simulink model "ciagly_zlinearyzowany_model_dynamiczny"  (R2022b)
settings: Solver=VariableStepAuto  StartTime=0.0  StopTime=100  RelTol=1e-3
values from neighbouring files (symbols this model uses):
  a0 = data.a0    [Projekt1.m]    (also in wykresy_char_stat_nlin.m; wykresy_char_stat_zlin.m)
  a1 = data.a1    [Projekt1.m]    (also in wykresy_char_stat_nlin.m; wykresy_char_stat_zlin.m)
  a2 = data.a2    [Projekt1.m]    (also in wykresy_char_stat_nlin.m; wykresy_char_stat_zlin.m)
  alpha1 = data.alpha1    [Projekt1.m]    (also in wykresy_char_stat_nlin.m; wykresy_char_stat_zlin.m)
  alpha2 = data.alpha2    [Projekt1.m]    (also in wykresy_char_stat_nlin.m; wykresy_char_stat_zlin.m)
  alpha3 = data.alpha3    [Projekt1.m]    (also in wykresy_char_stat_nlin.m; wykresy_char_stat_zlin.m)
  alpha4 = data.alpha4    [Projekt1.m]    (also in wykresy_char_stat_nlin.m; wykresy_char_stat_zlin.m)
  b0 = data.b0    [Projekt1.m]    (also in wykresy_char_stat_nlin.m; wykresy_char_stat_zlin.m)
  t_u_step_sim = 1    [wykresy_char_dyn_dys.m]    (also in wykresy_char_dyn_zlin.m)
  u_step_sim = 1    [wykresy_char_dyn_dys.m]    (also in wykresy_char_dyn_zlin.m = u_step(j))
  ud = uds(i)    [wykresy_char_dyn_zlin.m]
  X_0 = [0;0;0]    [Projekt1.m]
settings Model: Creator=pioro  LastModifiedBy=pioro

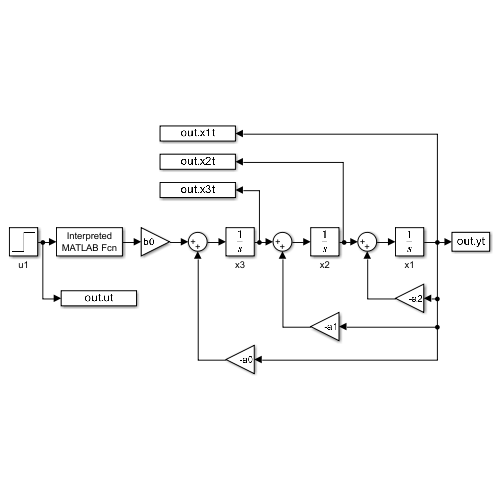
[thumbnail: Simulink's stored preview of the top-level diagram]
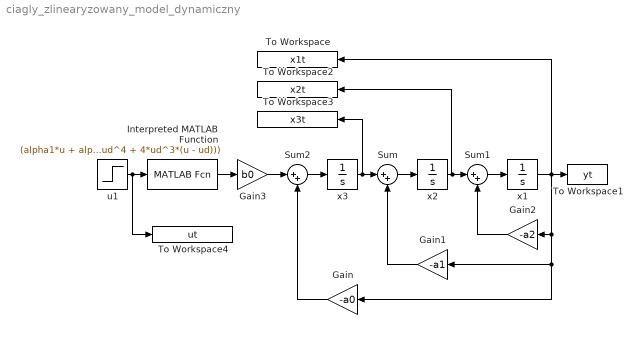
== system ciagly_zlinearyzowany_model_dynamiczny ==
  Gain : Gain  Gain=-a0
  Gain1 : Gain  Gain=-a1
  Gain2 : Gain  Gain=-a2
  Gain3 : Gain  Gain=b0
  Interpreted MATLAB Function : MATLABFcn  MATLABFcn=(alpha1*u + alpha2*(2*ud*(u - ud) + ud^2) + alpha3*(ud^3 + 3*ud^2*(u - ud)) + alpha4*(ud^4 + 4*ud^3*(u - ud)))
  Sum : Sum  Inputs=|++
  Sum1 : Sum  Inputs=|++
  Sum2 : Sum  Inputs=|++
  To Workspace : ToWorkspace  VariableName=x1t  SaveFormat=Timeseries  SampleTime=-1
  To Workspace1 : ToWorkspace  VariableName=yt  SaveFormat=Timeseries  SampleTime=-1
  To Workspace2 : ToWorkspace  VariableName=x2t  SaveFormat=Timeseries  SampleTime=-1
  To Workspace3 : ToWorkspace  VariableName=x3t  SaveFormat=Timeseries  SampleTime=-1
  To Workspace4 : ToWorkspace  VariableName=ut  SaveFormat=Timeseries  SampleTime=-1
  u1 : Step  Time=t_u_step_sim  After=u_step_sim  SampleTime=0
  x1 : Integrator  InitialCondition=X_0(1)
  x2 : Integrator  InitialCondition=X_0(2)
  x3 : Integrator  InitialCondition=X_0(3)
  wires:
  x3/1 -> To Workspace3/1, Sum/1
  x2/1 -> To Workspace2/1, Sum1/1
  Sum/1 -> x2/1
  Gain/1 -> Sum2/2
  Sum1/1 -> x1/1
  Gain3/1 -> Sum2/1
  Gain1/1 -> Sum/2
  Gain2/1 -> Sum1/2
  Interpreted MATLAB Function/1 -> Gain3/1
  Sum2/1 -> x3/1
  u1/1 -> To Workspace4/1, Interpreted MATLAB Function/1
  x1/1 -> To Workspace1/1, Gain2/1, Gain/1, Gain1/1, To Workspace/1
